simulink model "DC_Motor_PositionControl_CloseLoop"  (Simulink 7.3)
settings: Solver=ode45  StartTime=0.0  StopTime=10.0  RelTol=1e-3
values from neighbouring files (symbols this model uses):
  K = (Kt/Ra)*(1/(Kb+Beq))    (= 0.399201596806)    [Parameters.m]
  T = (Jeq/(Kb+Beq))    (= 0.499001996008)    [Parameters.m]
settings Model: Creator=ram  LastModifiedBy=ram

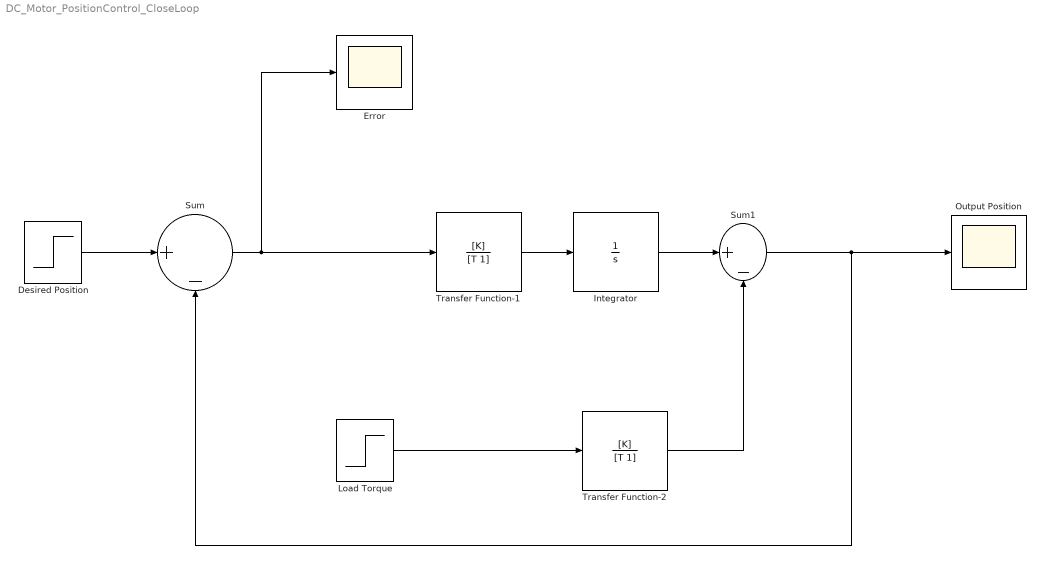
== system DC_Motor_PositionControl_CloseLoop ==
  Desired Position : Step  Time=0  After=5  SampleTime=0
  Error : Scope
  Integrator : TransferFcn  Denominator=[1 0]
  Load Torque : Step  Time=0  After=0  SampleTime=0
  Output Position : Scope
  Sum : Sum  Inputs=|+-  OutDataType=fixdt(1, 16)  OutScaling=2^0
  Sum1 : Sum  Inputs=|+-  OutDataType=fixdt(1, 16)  OutScaling=2^0
  Transfer Function-1 : TransferFcn  Numerator=[K]  Denominator=[T 1]
  Transfer Function-2 : TransferFcn  Numerator=[K]  Denominator=[T 1]
  wires:
  Transfer Function-1/1 -> Integrator/1
  Load Torque/1 -> Transfer Function-2/1
  Transfer Function-2/1 -> Sum1/2
  Sum1/1 -> Output Position/1, Sum/2
  Desired Position/1 -> Sum/1
  Integrator/1 -> Sum1/1
  Sum/1 -> Transfer Function-1/1, Error/1
